simulink model "Control_Pc"  (R2023b)
settings: Solver=FixedStepDiscrete  StartTime=0.0  StopTime=inf  FixedStep=0.01  MaxStep=0.01  RelTol=1e-3
InitFcn:
  | Ts=0.01;
libraries: instrumentseriallib x6, simulink x5
settings Model: Creator=eva_g  LastModifiedBy=merce
settings SolverCC: AlgebraicLoopSolver=TrustRegion
settings DebuggingCC: UnconnectedInputMsg=warning  UnconnectedOutputMsg=warning  UnconnectedLineMsg=warning
settings ModelReferenceCC: EnableRefExpFcnMdlSchedulingChecks=on
settings RTWCC: DLArmComputeVersion=19.05

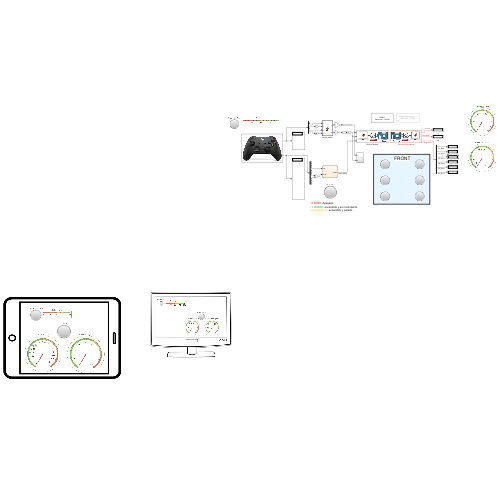
[thumbnail: Simulink's stored preview of the top-level diagram]
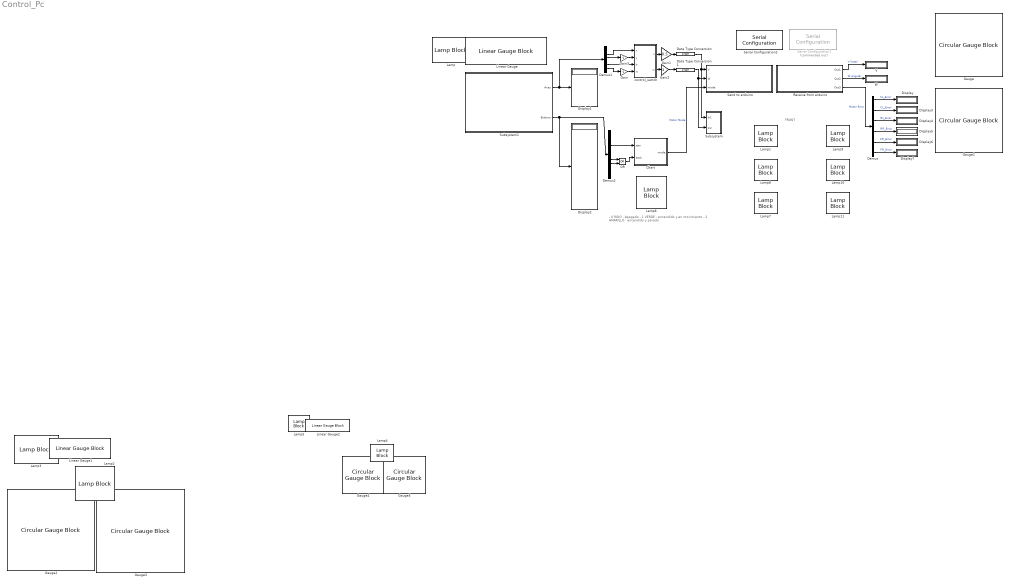
== system Control_Pc ==
  note: FRONT
  note: - 0 ROJO : Apagado
      | - 1 VERDE : encendido y en movimiento
      | - 2 AMARILLO : encendido y parado
  Chart : Stateflow chart  TreatAsAtomicUnit=on
  Data Type Conversion : DataTypeConversion  OutDataTypeStr=single  SaturateOnIntegerOverflow=off  RndMeth=Floor
  Data Type Conversion1 : DataTypeConversion  OutDataTypeStr=single  SaturateOnIntegerOverflow=off  RndMeth=Floor
  Demux : Demux  Outputs=6
  Demux1 : Demux  Outputs=6
  Demux2 : Demux  Outputs=14
  Display{,1..7} (8 alike) : Display
  Gain : Gain  Gain=-1
  Gain1 : Gain  Gain=0.5
  Gain2 : Gain
  Gain3 : Gain  Gain=-1
  Gauge : CircularGaugeBlock  ScaleMax=2
  Gauge1 : CircularGaugeBlock  ScaleMax=1.2
  Gauge2 : CircularGaugeBlock  ScaleMax=2
  Gauge3 : CircularGaugeBlock  ScaleMax=1.2
  Gauge4 : CircularGaugeBlock  ScaleMax=2
  Gauge5 : CircularGaugeBlock  ScaleMax=1.2
  Lamp{,2..6} (6 alike) : LampBlock
  Lamp{1,7..11} (6 alike) : LampBlock  LabelPosition=Hide
  Linear Gauge : LinearGaugeBlock  TickInterval=25
  Linear Gauge1 : LinearGaugeBlock  TickInterval=25
  Linear Gauge2 : LinearGaugeBlock  TickInterval=25
  OR : Logic  Operator=OR  IconShape=distinctive  AllPortsSameDT=off  OutDataTypeStr=boolean
  Receive from arduino : Subsystem
      mask Display: image('am.jpg'); % Use "Edit Image" on toolstrip to change.
  Send to arduino : Subsystem
      mask Display: image('ma.jpg'); % Use "Edit Image" on toolstrip to change.
  Serial Configuration1 : instrumentseriallib/Serial Configuration  Priority=-200000  Commented=on  PortSel=<Please select a port...>  Port=<Select a port...>  ComPort=COM5  BaudRate=115200  DataBits=8  Parity=none  StopBits=1  ByteOrder=little-endian  FlowControl=none  Timeout=10  SimulateUsing=Interpreted execution  BlockInModel=on  aMode=1
  Serial Configuration2 : instrumentseriallib/Serial Configuration  Priority=-200000  PortSel=COM11  Port=COM11  ComPort=COM11  BaudRate=115200  DataBits=8  Parity=none  StopBits=1  ByteOrder=little-endian  FlowControl=none  Timeout=10  SimulateUsing=Interpreted execution  BlockInModel=on  aMode=1
  Subsystem : Subsystem
  Subsystem1 : Subsystem
      mask Display: image('mando.PNG'); % Use "Edit Image" on toolstrip to change.
  V : Display
  W : Display
  control_switch : MATLAB Function  TreatAsAtomicUnit=on
  wires:
  Demux2/9 -> OR/1
  Gain1/1 -> Data Type Conversion/1
  Demux2/10 -> OR/2
  control_switch/1(v) -> Gain1/1
  Demux1/2 -> control_switch/1(x)
  Gain3/1 -> control_switch/2(y)
  control_switch/2(w) -> Gain2/1
  Demux2/5 -> Chart/1(star)
  Gain/1 -> control_switch/4(rt)
  Receive from arduino/3(Out3) -> Demux/1  "Motor Error"
  Chart/1(mode) -> Send to arduino/3(mode)  "Motor Mode"
  Demux1/3 -> Gain3/1
  Receive from arduino/2(Out2) -> W/1  "W angular"
  Gain2/1 -> Data Type Conversion1/1
  OR/1 -> Chart/2(back)
  Demux1/6 -> Gain/1
  Demux1/5 -> control_switch/3(lt)
  Receive from arduino/1(Out1) -> V/1  "V lineal"
  Data Type Conversion/1 -> Subsystem/1(In1), Send to arduino/1(V)
  Data Type Conversion1/1 -> Send to arduino/2(W), Subsystem/2(In2)
  Subsystem1/2(Buttons) -> Display2/1, Demux2/1
  Subsystem1/1(Axes) -> Display1/1, Demux1/1
  Demux/1 -> Display/1  "FL_Error"
  Demux/2 -> Display3/1  "CL_Error"
  Demux/3 -> Display4/1  "RL_Error"
  Demux/4 -> Display5/1  "RR_Error"
  Demux/5 -> Display6/1  "CR_Error"
  Demux/6 -> Display7/1  "FR_Error"

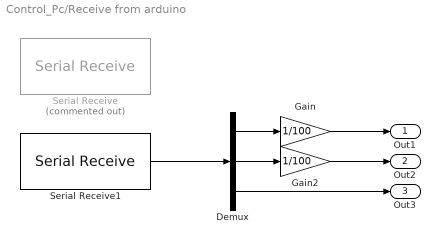
== system Control_Pc/Receive from arduino ==
  Demux : Demux  Outputs=3
  Gain : Gain  Gain=1/100
  Gain2 : Gain  Gain=1/100
  Serial Receive : instrumentseriallib/Serial Receive  Commented=on  PortSel=<Select a port...>  Port=<Select a port...>  ComPort=COM5  DataType=int16  SaveDataType=uint8  ToggleHeader=off  Header=[]  ToggleTerminator=on  Terminator=<none>  CustomTerminator=[]  InputFormat=Column major  ToggleDataSize=on  DataSize="[1  3]"  EnableBlockingMode=on  ActionDataUnavailable=Output last received value  ActionWhenDataUnavailable=Output last received value  CustomValue=0  SampleTime=Ts  SimulateUsing=Interpreted execution  BlockInModel=on  aMode=1
  Serial Receive1 : instrumentseriallib/Serial Receive  PortSel=COM11  Port=COM11  ComPort=COM11  DataType=int16  SaveDataType=uint8  ToggleHeader=off  Header=[]  ToggleTerminator=on  Terminator=<none>  CustomTerminator=[]  InputFormat=Column major  ToggleDataSize=on  DataSize="[1  3]"  EnableBlockingMode=on  ActionDataUnavailable=Output last received value  ActionWhenDataUnavailable=Output last received value  CustomValue=0  SampleTime=0.01  SimulateUsing=Interpreted execution  BlockInModel=on  aMode=1
  Out1 : Outport
  Out2 : Outport  Port=2
  Out3 : Outport  Port=3
  wires:
  Gain/1 -> Out1/1
  Demux/1 -> Gain/1
  Gain2/1 -> Out2/1
  Demux/2 -> Gain2/1
  Demux/3 -> Out3/1
  Serial Receive1/1 -> Demux/1

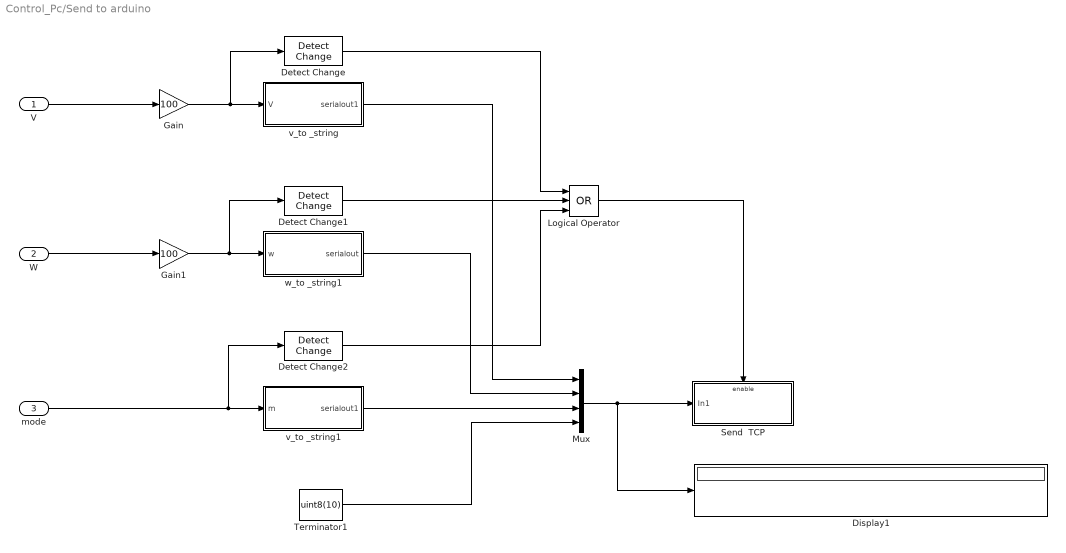
== system Control_Pc/Send to arduino ==
  V : Inport
  W : Inport  Port=2
  mode : Inport  Port=3
  Detect Change : simulink/Logic and Bit Operations/Detect Change  vinit=0  OutDataTypeStr=boolean
  Detect Change1 : simulink/Logic and Bit Operations/Detect Change  vinit=0  OutDataTypeStr=boolean
  Detect Change2 : simulink/Logic and Bit Operations/Detect Change  vinit=0  OutDataTypeStr=boolean
  Display1 : Display
  Gain : Gain  Gain=100
  Gain1 : Gain  Gain=100
  Logical Operator : Logic  Operator=OR  Inputs=3  AllPortsSameDT=off  OutDataTypeStr=boolean
  Mux : Mux
  Send  TCP : Subsystem  TreatAsAtomicUnit=on
  Terminator1 : Constant  Value=uint8(10)
  v_to _string : Subsystem
  v_to _string1 : Subsystem
  w_to _string1 : Subsystem
  wires:
  Detect Change/1 -> Logical Operator/1
  Gain/1 -> v_to _string/1(V), Detect Change/1
  Detect Change1/1 -> Logical Operator/2
  Mux/1 -> Display1/1, Send  TCP/1(In1)
  W/1 -> Gain1/1
  V/1 -> Gain/1
  Gain1/1 -> Detect Change1/1, w_to _string1/1(w)
  v_to _string/1(serialout1) -> Mux/1
  w_to _string1/1(serialout) -> Mux/2
  Logical Operator/1 -> Send  TCP/Enable
  v_to _string1/1(serialout1) -> Mux/3
  mode/1 -> v_to _string1/1(m), Detect Change2/1
  Terminator1/1 -> Mux/4
  Detect Change2/1 -> Logical Operator/3

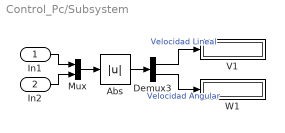
== system Control_Pc/Subsystem ==
  In1 : Inport
  In2 : Inport  Port=2
  Abs : Abs  SaturateOnIntegerOverflow=off
  Demux3 : Demux  Outputs=2
  Mux : Mux  Inputs=2
  V1 : Display
  W1 : Display
  wires:
  Demux3/1 -> V1/1  "Velocidad Lineal"
  Mux/1 -> Abs/1
  Abs/1 -> Demux3/1
  In1/1 -> Mux/1
  Demux3/2 -> W1/1  "Velocidad Angular"
  In2/1 -> Mux/2

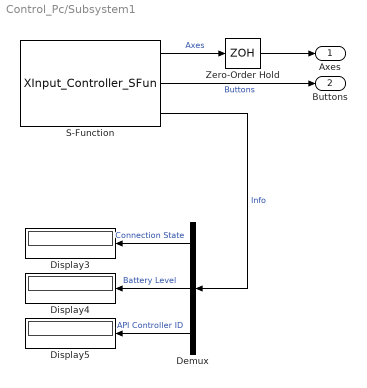
== system Control_Pc/Subsystem1 ==
  Demux : Demux  Outputs=3
  Display3 : Display
  Display4 : Display
  Display5 : Display
  S-Function : S-Function  FunctionName=XInput_Controller_SFun  Parameters=ControllerID  SFunctionDeploymentMode=off  EnableBusSupport=off  mask(XInput Controller){ControllerID=1}
      mask help:
      | This Block will allow you to use XInput Controllers in Simulink.
      | XInput is the most Supported API.
      | Works with XBOX 360 and XBOX ONE Controllers.
      |
      | Use 'DEMUX' to access Signals
      | Output_1 [1x6]
      |   Analog Left X, Analog Left Y,
      |   Analog Right X, Analog Right Y,
      |   Left Trigger, Right Trigger
      | Output_2 [1x14]
      |   Up, Down, Left, Right,
      |   Start, Back, Left Stick, Right Stick,
      |   Left Shoulder, Right Shoulder,
      |   A, B, X, Y
      | Output_3 [1x3]
      |   Connection State, Battery Level (1-4), Controller ID
      mask init:
      | ControllerID;   
      | blk = gcb; 
      | get_String = get_param(blk,'ControllerID');
      | ControllerID = str2double(get_String);
      mask Help:
      | Based on Microsoft XInput API
      | Therefore the maximum of conneced Gamepads per PC is 4. First Gamepad has Controller ID 1.
      | 
      | Reference:
      | https://docs.microsoft.com/en-us/windows/win32/api/_xinput/
      | 
      | Tutorial:
      | https://docs.microsoft.com/en-us/windows/win32/xinput/getting-started-with-xinput
      | 
      | Info:
      | The Analog Sticks Deadzone is coded to:
      | Deadzone = 6144;
      | 0 <= Deadzone <= 65534
      | This is smaller then Microsoft default.
      | 
      | created by Mathias Voigt
      | Technische Universität Dresden
      | 2019
      mask TypeOptions ControllerID: 1 | 2 | 3 | 4
      mask DialogControl ParameterGroupVar Prompt: Controller ID
      mask Display:
      | %% Set Block picture from user Data
      | %  (permanent, picture file not needed)
      | %  see persistent_image_allocation.m
      | 
      | %get the picture data
      | UserDataStrut = get_param(gcb, 'UserData');
      | image(UserDataStrut.Image, [0.2, 0.3, 0.6, 0.6])
      | 
      | 
      | 
      | % conventional method (does not save picture data in Simulink)
      | % image('XBOX_One_Controller_Icon.png', [0.2, 0.3, 0.6, 0.6])
      | 
      | %% Create Port Labels
      | color('blue');
      | port_label('output', 1, 'Axes');
      | port_label('output', 2, 'Buttons');
      | port_label('output', 3, 'Info');
      | 
      | 
      | %% Create S-Function Block Name
      | color('black');
      | text(0.5, 0.1, 'XInput Controller',...
      |      'horizontalAlignment', 'center',...
      |      'verticalAlignment', 'bottom');
  Zero-Order Hold : ZeroOrderHold  SampleTime=-1
  Axes : Outport
  Buttons : Outport  Port=2
  wires:
  Demux/1 -> Display3/1  "Connection State"
  Demux/2 -> Display4/1  "Battery Level"
  Zero-Order Hold/1 -> Axes/1
  Demux/3 -> Display5/1  "API Controller ID"
  S-Function/1 -> Zero-Order Hold/1  "Axes"
  S-Function/3 -> Demux/1  "Info"
  S-Function/2 -> Buttons/1  "Buttons"

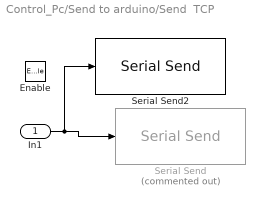
== system Control_Pc/Send to arduino/Send  TCP ==
  In1 : Inport
  Enable : EnablePort
  Serial Send : instrumentseriallib/Serial Send  Commented=on  PortSel=COM11  Port=COM11  ComPort=COM11  Header=[]  Terminator=<none>  CustomTerminator=[]  EnableBlockingMode=on  SimulateUsing=Interpreted execution  BlockInModel=on  aMode=1
  Serial Send2 : instrumentseriallib/Serial Send  PortSel=COM11  Port=COM11  ComPort=COM11  Header=[]  Terminator=<none>  CustomTerminator=[]  EnableBlockingMode=on  SimulateUsing=Interpreted execution  BlockInModel=on  aMode=1
  wires:
  In1/1 -> Serial Send2/1, Serial Send/1

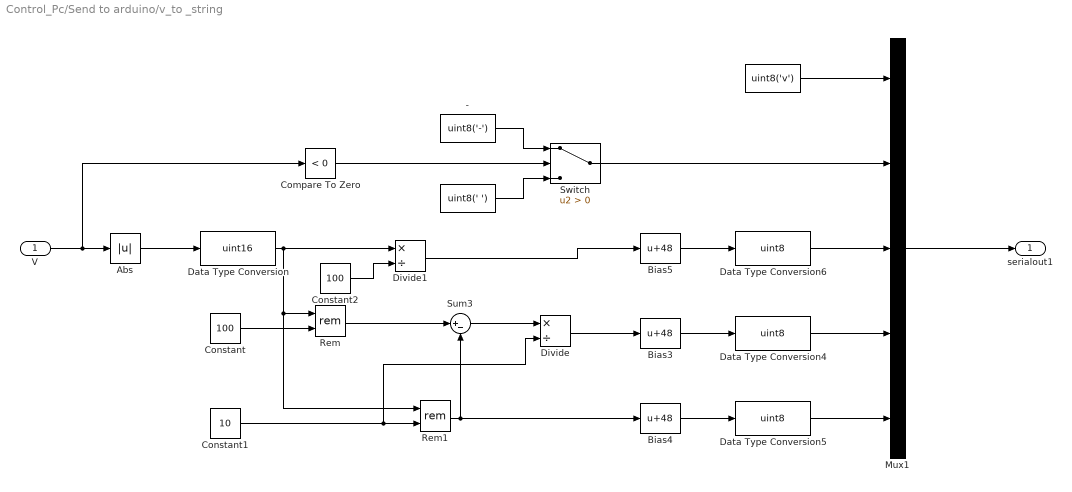
== system Control_Pc/Send to arduino/v_to _string ==
  V : Inport
  "     " : Constant  Value=uint8(' ')
  "       " : Constant  Value=uint8('v')
  "  -" : Constant  Value=uint8('-')
  Abs : Abs  SaturateOnIntegerOverflow=off
  Bias3 : Bias  Bias=48  SaturateOnIntegerOverflow=off
  Bias4 : Bias  Bias=48  SaturateOnIntegerOverflow=off
  Bias5 : Bias  Bias=48  SaturateOnIntegerOverflow=off
  Compare To Zero : simulink/Logic and Bit Operations/Compare To Zero  relop=<  OutDataTypeStr=boolean
  Constant : Constant  Value=100  OutDataTypeStr=uint16
  Constant1 : Constant  Value=10  OutDataTypeStr=uint16
  Constant2 : Constant  Value=100  OutDataTypeStr=uint16
  Data Type Conversion : DataTypeConversion  OutDataTypeStr=uint16  SaturateOnIntegerOverflow=off  RndMeth=Floor
  Data Type Conversion4 : DataTypeConversion  OutDataTypeStr=uint8  SaturateOnIntegerOverflow=off  RndMeth=Floor
  Data Type Conversion5 : DataTypeConversion  OutDataTypeStr=uint8  SaturateOnIntegerOverflow=off  RndMeth=Floor
  Data Type Conversion6 : DataTypeConversion  OutDataTypeStr=uint8  SaturateOnIntegerOverflow=off  RndMeth=Floor
  Divide : Product  Inputs=*/
  Divide1 : Product  Inputs=*/
  Mux1 : Mux  Inputs=5
  Rem : Math  Operator=rem
  Rem1 : Math  Operator=rem
  Sum3 : Sum  Inputs=|+-
  Switch : Switch  Criteria=u2 > Threshold  SaturateOnIntegerOverflow=off  InputSameDT=off
  serialout1 : Outport
  wires:
  Divide1/1 -> Bias5/1
  V/1 -> Compare To Zero/1, Abs/1
  Bias5/1 -> Data Type Conversion6/1
  Bias4/1 -> Data Type Conversion5/1
  Bias3/1 -> Data Type Conversion4/1
  Mux1/1 -> serialout1/1
  "       "/1 -> Mux1/1
  Data Type Conversion5/1 -> Mux1/5
  Data Type Conversion4/1 -> Mux1/4
  Data Type Conversion6/1 -> Mux1/3
  Compare To Zero/1 -> Switch/2
  "     "/1 -> Switch/3
  "  -"/1 -> Switch/1
  Switch/1 -> Mux1/2
  Constant/1 -> Rem/2
  Sum3/1 -> Divide/1
  Rem/1 -> Sum3/1
  Constant1/1 -> Divide/2, Rem1/2
  Abs/1 -> Data Type Conversion/1
  Rem1/1 -> Bias4/1, Sum3/2
  Divide/1 -> Bias3/1
  Data Type Conversion/1 -> Divide1/1, Rem1/1, Rem/1
  Constant2/1 -> Divide1/2

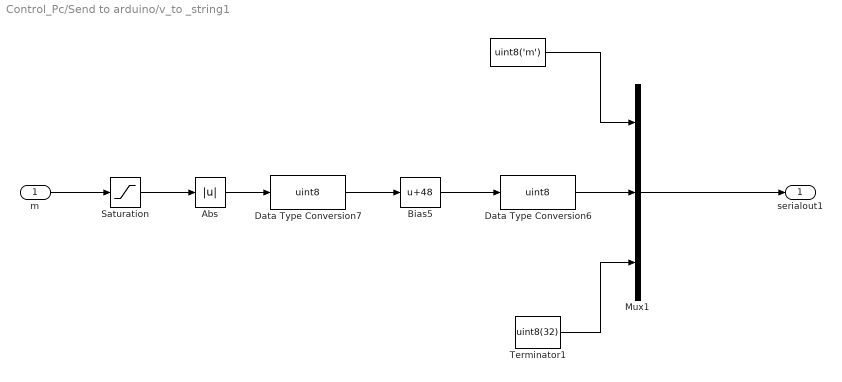
== system Control_Pc/Send to arduino/v_to _string1 ==
  m : Inport
  "       " : Constant  Value=uint8('m')
  Abs : Abs  SaturateOnIntegerOverflow=off
  Bias5 : Bias  Bias=48  SaturateOnIntegerOverflow=off
  Data Type Conversion6 : DataTypeConversion  OutDataTypeStr=uint8  SaturateOnIntegerOverflow=off  RndMeth=Floor
  Data Type Conversion7 : DataTypeConversion  OutDataTypeStr=uint8  SaturateOnIntegerOverflow=off  RndMeth=Floor
  Mux1 : Mux  Inputs=3
  Saturation : Saturate  UpperLimit=1  LowerLimit=0
  Terminator1 : Constant  Value=uint8(32)
  serialout1 : Outport
  wires:
  Abs/1 -> Data Type Conversion7/1
  Data Type Conversion6/1 -> Mux1/2
  Terminator1/1 -> Mux1/3
  "       "/1 -> Mux1/1
  Mux1/1 -> serialout1/1
  Data Type Conversion7/1 -> Bias5/1
  Bias5/1 -> Data Type Conversion6/1
  m/1 -> Saturation/1
  Saturation/1 -> Abs/1

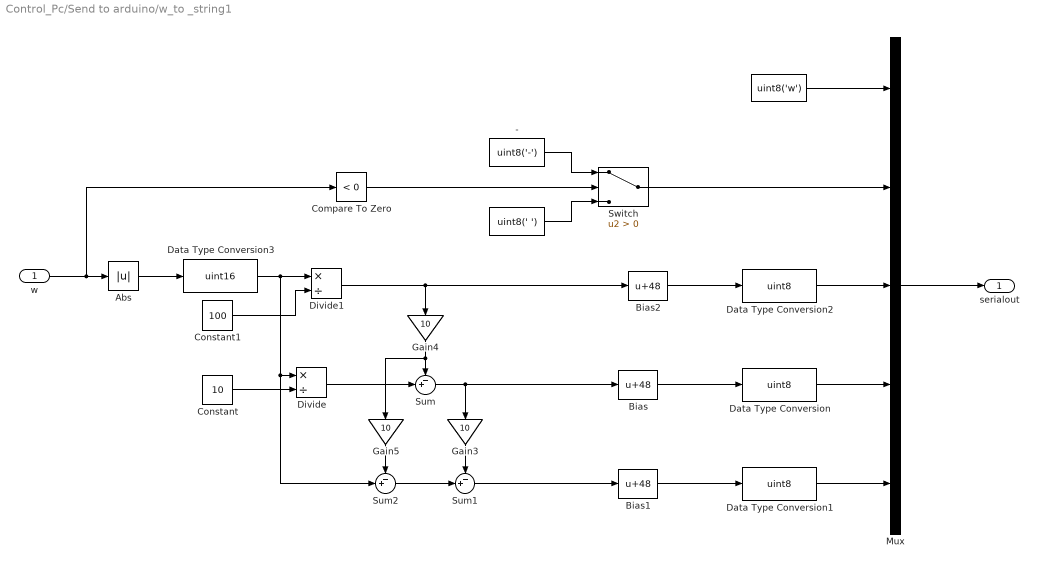
== system Control_Pc/Send to arduino/w_to _string1 ==
  w : Inport
  "  " : Constant  Value=uint8('w')
  "     " : Constant  Value=uint8(' ')
  "  -" : Constant  Value=uint8('-')
  Abs : Abs  SaturateOnIntegerOverflow=off
  Bias : Bias  Bias=48  SaturateOnIntegerOverflow=off
  Bias1 : Bias  Bias=48  SaturateOnIntegerOverflow=off
  Bias2 : Bias  Bias=48  SaturateOnIntegerOverflow=off
  Compare To Zero : simulink/Logic and Bit Operations/Compare To Zero  relop=<  OutDataTypeStr=boolean
  Constant : Constant  Value=10  OutDataTypeStr=int16
  Constant1 : Constant  Value=100  OutDataTypeStr=int16
  Data Type Conversion : DataTypeConversion  OutDataTypeStr=uint8  SaturateOnIntegerOverflow=off  RndMeth=Floor
  Data Type Conversion1 : DataTypeConversion  OutDataTypeStr=uint8  SaturateOnIntegerOverflow=off  RndMeth=Floor
  Data Type Conversion2 : DataTypeConversion  OutDataTypeStr=uint8  SaturateOnIntegerOverflow=off  RndMeth=Floor
  Data Type Conversion3 : DataTypeConversion  OutDataTypeStr=uint16  SaturateOnIntegerOverflow=off  RndMeth=Floor
  Divide : Product  Inputs=*/
  Divide1 : Product  Inputs=*/
  Gain3 : Gain  Gain=10
  Gain4 : Gain  Gain=10
  Gain5 : Gain  Gain=10
  Mux : Mux  Inputs=5
  Sum : Sum  Inputs=-+|
  Sum1 : Sum  Inputs=-+|
  Sum2 : Sum  Inputs=-+|
  Switch : Switch  Criteria=u2 > Threshold  SaturateOnIntegerOverflow=off  InputSameDT=off
  serialout : Outport  OutDataTypeStr=uint8
  wires:
  Sum1/1 -> Bias1/1
  Gain5/1 -> Sum2/1
  Sum2/1 -> Sum1/2
  Gain3/1 -> Sum1/1
  Gain4/1 -> Gain5/1, Sum/1
  Sum/1 -> Bias/1, Gain3/1
  Divide/1 -> Sum/2
  Data Type Conversion3/1 -> Sum2/2, Divide/1, Divide1/1
  w/1 -> Compare To Zero/1, Abs/1
  Bias2/1 -> Data Type Conversion2/1
  Divide1/1 -> Bias2/1, Gain4/1
  Bias1/1 -> Data Type Conversion1/1
  Bias/1 -> Data Type Conversion/1
  Mux/1 -> serialout/1
  "  "/1 -> Mux/1
  Data Type Conversion1/1 -> Mux/5
  Data Type Conversion/1 -> Mux/4
  Data Type Conversion2/1 -> Mux/3
  Compare To Zero/1 -> Switch/2
  "     "/1 -> Switch/3
  "  -"/1 -> Switch/1
  Switch/1 -> Mux/2
  Abs/1 -> Data Type Conversion3/1
  Constant/1 -> Divide/2
  Constant1/1 -> Divide1/2

== stateflow chart Control_Pc/Chart ==
  state ON
    entry: mode=1;
  state OFF
    entry: mode=0;
  (default) -> OFF
  ON -> OFF : [back>0]
  OFF -> ON : [star>0]
  data: mode output; star input; back input

== matlab function Control_Pc/control_switch ==
  data: x input; v output; y input; lt input; rt input; w output
function [v,w]=fcn(x,y,lt,rt)

    if (rt==0) && (lt==0) && ((x>=0.3) || (x<=-0.3))
        v=x;
        w=y;
    elseif (x~=0) && ((rt~=0) || (lt~=0))
        w=0;
        v=0;
    elseif (x==0) && (y==0) && (rt==0) && (lt~=0)
        w=lt;
        v=0;
    elseif (x==0) && (y==0) && (lt==0) && (rt~=0)
        w=rt;
        v=0;
    elseif (lt~=0) && (rt~=0)
        w=0;
        v=0;
    elseif (x==0) || (y==0) || (lt==0) 
        w=lt;
        v=0;
    else
        w=0;
        v=0;
    end;
